simulink model "P1_DevDriv_z_krancowka_2015a"  (R2020b)
settings: Solver=ode5  StartTime=0.0  StopTime=999  FixedStep=0.01  RelTol=1e-3  AbsTol=1e-6
undefined symbols (not defined in the file): Cntrl, K_reg, RTDAC4PCIBaseAddress, x_konc
libraries: simulink x2
settings Model: SimulationMode=external  ExtModeTrigDuration=12000  ExtModeTrigDurationFloating=999000  ExtModeTrigLevel=0.400000  Creator=jims  LastModifiedBy=maelstro
settings SolverCC: AutoScaleAbsTol=off
settings DataIOCC: ExternalInput=[]  InitialState=[]  MaxDataPoints=5000  SaveFormat=Array  SignalLoggingSaveFormat=ModelDataLogs  SaveOutput=off  SaveTime=off  ReturnWorkspaceOutputs=off  SignalLoggingName=sigsOut
settings OptimizationCC: BooleanDataType=off  ExpressionDepthLimit=2147483647  LifeSpan=inf
settings DebuggingCC: SaveWithParameterizedLinksMsg=none  UnderspecifiedInitializationDetection=Classic  MergeDetectMultiDrivingBlocksExec=none  SignalResolutionControl=TryResolveAllWithWarning  MultiTaskDSMMsg=warning  MultiTaskCondExecSysMsg=none  IntegerOverflowMsg=none  FcnCallInpInsideContextMsg=warning  StateNameClashWarn=warning  SFUnexpectedBacktrackingDiag=warning  SFNoUnconditionalDefaultTransitionDiag=warning  SFExecutionAtInitializationDiag=none  IntegerSaturationMsg=none  ArithmeticOperatorsInVariantConditions=warning
settings HardwareCC: ProdBitPerLong=64  ProdLargestAtomicFloat=None  ProdHWDeviceType=Intel->x86-64  TargetBitPerLong=64  TargetBitPerPointer=64  TargetIntDivRoundTo=Zero  TargetEndianess=LittleEndian  TargetWordSize=64  TargetHWDeviceType=Intel->x86-64
settings ModelReferenceCC: PropagateSignalLabelsOutOfModel=off
settings SFSimCC: SimUseLocalCustomCode=off  CustomCodeUndefinedFunction=UseInterfaceOnly
settings RTWCC: Description=Real-Time Windows Target  SystemTargetFile=rtwin.tlc  TemplateMakefile=rtwin.tmf  RTWUseLocalCustomCode=off  RTWCompilerOptimization=on
settings CodeAppCC: MaxIdLength=95  StateflowObjectComments=on
settings TargetCC: TargetPreCompLibLocation=C:\Program Files\MATLAB\R2015aSP1\toolbox\sldrt\lib\win64
settings ConfigComp: CovMetricSettings=dw  CovSaveCumulativeToWorkspaceVar=on  CovSaveSingleToWorkspaceVar=on  CovExternalEMLEnable=off  CovSFcnEnable=off

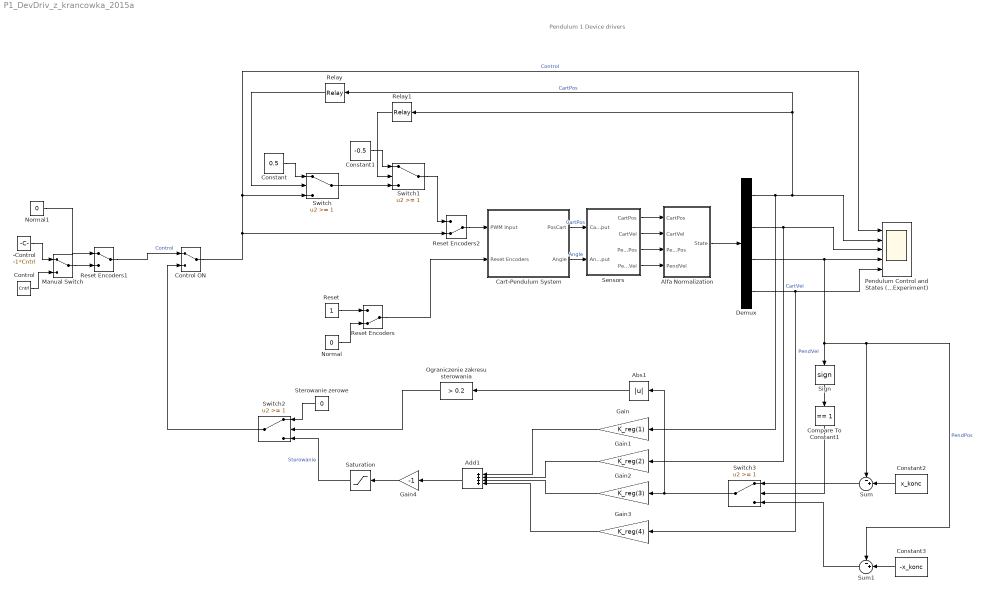
== system P1_DevDriv_z_krancowka_2015a ==
  note: Pendulum 1
      | Device drivers
  -Control : Constant  Value=-1*Cntrl
  Abs1 : Abs
  Add1 : Sum  Inputs=++++
  Alfa Normalization : Subsystem  mask(Choose mode:){pos=Crane Controller}
      mask prompts: pos "Choose mode:"
      mask TypeOptions pos: Inverted Pendulum | Crane Controller
  Cart-Pendulum System : Subsystem  mask{BaseAddress=RTDAC4PCIBaseAddress(-1,-1), T0=0.01}
      mask prompts: BaseAddress "Base Address:"; T0 "Sampling Period:"
      mask Display: plot( [0.725 0.725], [1.05 0.375], 0.725+0.05*sin([0:0.5:7]), 0.325+0.05*cos([0:0.5:7]), [-0.3 -0.3], [-0.3 -0.3], [1.8 1.8], [1.8 1.8], [0.1 1.4], [0.95 0.95], [0.1 1.4], [0.92 0.92], [0.65 0.8], [1 1], [0.65 0.8], [1.1 1.1], [0.65 0.65], [1.1 1], [0.8 0.8], [1 1.1] )
  Compare To Constant1 : simulink/Logic and Bit Operations/Compare To Constant  relop===  const=1  OutDataTypeStr=boolean
  Constant : Constant  Value=0.5
  Constant1 : Constant  Value=-0.5
  Constant2 : Constant  Value=x_konc
  Constant3 : Constant  Value=-x_konc
  Control : Constant  Value=Cntrl
  Control ON : ManualSwitch
  Demux : Demux
      settings: DisplayOption=none
  Gain : Gain  Gain=K_reg(1)
  Gain1 : Gain  Gain=K_reg(2)
  Gain2 : Gain  Gain=K_reg(3)
  Gain3 : Gain  Gain=K_reg(4)
  Gain4 : Gain  Gain=-1
  Manual Switch : ManualSwitch
  Normal : Constant  Value=0
  Normal1 : Constant  Value=0
  Ograniczenie zakresu sterowania : simulink/Logic and Bit Operations/Compare To Constant  relop=>  const=0.2  OutDataTypeStr=boolean
  Pendulum Control and States (Experiment) : Scope  NumInputPorts=5
  Relay : Relay  OnSwitchValue=0.7  OffSwitchValue=0.6
  Relay1 : Relay  OnSwitchValue=-0.6  OffSwitchValue=-0.7  OnOutputValue=0  OffOutputValue=1
  Reset : Constant
  Reset Encoders : ManualSwitch  CurrentSetting=0
  Reset Encoders1 : ManualSwitch
  Reset Encoders2 : ManualSwitch  CurrentSetting=0
  Saturation : Saturate  UpperLimit=1  LowerLimit=-1
  Sensors : Subsystem  mask(PENDULUM Output){T0=0.01}
      mask prompts: T0 "Sample Time"
      mask help: PCL-812 PG Device Driver
  Sign : Signum
  Sterowanie zerowe : Constant  Value=0
  Sum : Sum  Inputs=-+|
  Sum1 : Sum  Inputs=-+|
  Switch{,1..3} (4 alike) : Switch  Threshold=1
  wires:
  Reset Encoders/1 -> Cart-Pendulum System/2(Reset Encoders)
  Sensors/3(PendPos) -> Alfa Normalization/3(PendPos)
  Sensors/4(PendVel) -> Alfa Normalization/4(PendVel)
  Sensors/1(CartPos) -> Alfa Normalization/1(CartPos)
  Sensors/2(CartVel) -> Alfa Normalization/2(CartVel)
  Demux/1 -> Gain/1, Pendulum Control and States (Experiment)/2, Relay/1, Relay1/1  "CartPos"
  Demux/2 -> Gain1/1, Pendulum Control and States (Experiment)/3  "CartVel"
  Demux/3 -> Sum1/1, Sum/1, Sign/1, Pendulum Control and States (Experiment)/4  "PendPos"
  Demux/4 -> Gain3/1, Pendulum Control and States (Experiment)/5  "PendVel"
  Cart-Pendulum System/1(PosCart) -> Sensors/1(CartPosInput)  "CartPos"
  Cart-Pendulum System/2(Angle) -> Sensors/2(AngleInput)  "Angle"
  Normal/1 -> Reset Encoders/2
  Reset/1 -> Reset Encoders/1
  Normal1/1 -> Reset Encoders1/1
  Manual Switch/1 -> Reset Encoders1/2
  Control/1 -> Manual Switch/2
  -Control/1 -> Manual Switch/1
  Control ON/1 -> Reset Encoders2/2, Pendulum Control and States (Experiment)/1, Switch/3  "Control"
  Relay/1 -> Switch/2
  Constant/1 -> Switch/1
  Reset Encoders2/1 -> Cart-Pendulum System/1(PWM Input)
  Relay1/1 -> Switch1/2
  Constant1/1 -> Switch1/1
  Switch/1 -> Switch1/3
  Switch1/1 -> Reset Encoders2/1
  Gain/1 -> Add1/1
  Gain1/1 -> Add1/2
  Gain2/1 -> Add1/3
  Gain3/1 -> Add1/4
  Constant2/1 -> Sum/2
  Add1/1 -> Gain4/1
  Gain4/1 -> Saturation/1
  Reset Encoders1/1 -> Control ON/1  "Control"
  Abs1/1 -> Ograniczenie zakresu sterowania/1
  Ograniczenie zakresu sterowania/1 -> Switch2/2
  Sterowanie zerowe/1 -> Switch2/1
  Saturation/1 -> Switch2/3  "Sterowanie"
  Switch2/1 -> Control ON/2
  Constant3/1 -> Sum1/2
  Sign/1 -> Compare To Constant1/1
  Compare To Constant1/1 -> Switch3/2
  Sum/1 -> Switch3/1
  Sum1/1 -> Switch3/3
  Alfa Normalization/1(State) -> Demux/1
  Switch3/1 -> Gain2/1, Abs1/1

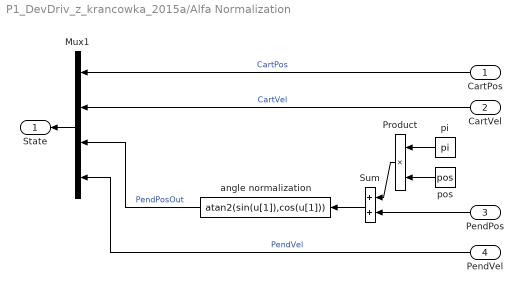
== system P1_DevDriv_z_krancowka_2015a/Alfa Normalization ==
  CartPos : Inport
  CartVel : Inport  Port=2
  PendPos : Inport  Port=3
  PendVel : Inport  Port=4
  Mux1 : Mux
  Product : Product  InputSameDT=on  SaturateOnIntegerOverflow=on  OutDataTypeStr=Inherit: Same as first input
  Sum : Sum  InputSameDT=on  SaturateOnIntegerOverflow=on  OutDataTypeStr=Inherit: Same as first input
  angle normalization : Fcn  Expr=atan2(sin(u[1]),cos(u[1]))
  pi : Constant  Value=pi
  pos : Constant  Value=pos
  State : Outport  InitialOutput=0
  wires:
  angle normalization/1 -> Mux1/3  "PendPosOut"
  PendVel/1 -> Mux1/4  "PendVel"
  CartVel/1 -> Mux1/2  "CartVel"
  CartPos/1 -> Mux1/1  "CartPos"
  Mux1/1 -> State/1
  Sum/1 -> angle normalization/1
  PendPos/1 -> Sum/2
  pi/1 -> Product/1
  pos/1 -> Product/2
  Product/1 -> Sum/1

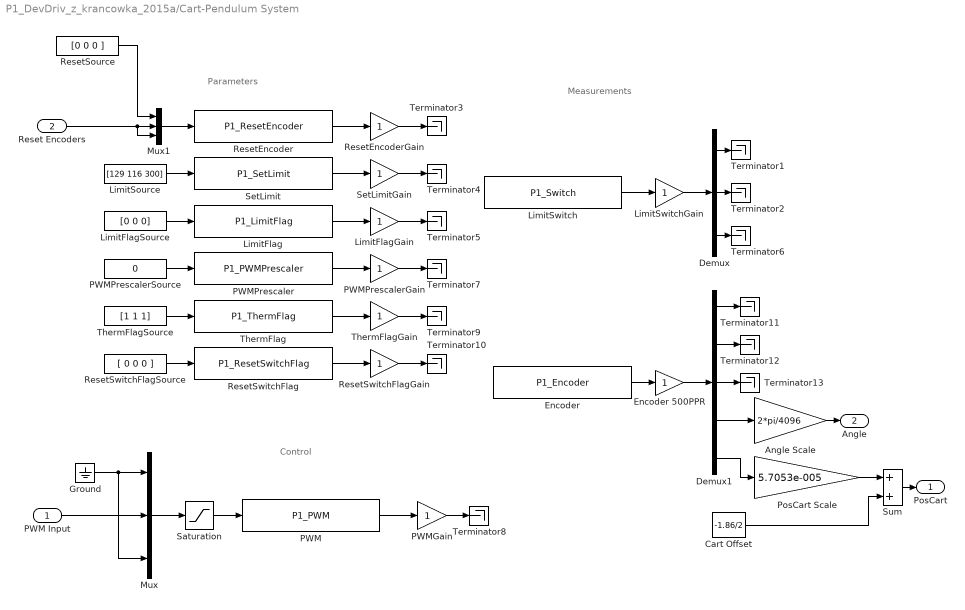
== system P1_DevDriv_z_krancowka_2015a/Cart-Pendulum System ==
  note: Measurements
  note: Control
  note: Parameters
  PWM Input : Inport
  Reset Encoders : Inport  Port=2
  Angle Scale : Gain  Gain=2*pi/4096  OutDataTypeStr=Inherit: Same as input  ParamDataTypeStr=Inherit: Same as input
  Cart Offset : Constant  Value=-1.86/2
  Demux : Demux  Outputs=3
      settings: DisplayOption=none
  Demux1 : Demux  Outputs=5
      settings: DisplayOption=none
  Encoder : S-Function  FunctionName=P1_Encoder  Parameters=BaseAddress, T0  SFunctionDeploymentMode=off  EnableBusSupport=off
  Encoder 500PPR : Gain  SaturateOnIntegerOverflow=on  OutDataTypeStr=Inherit: Same as input  ParamDataTypeStr=Inherit: Same as input
  Ground : Ground
  LimitFlag : S-Function  FunctionName=P1_LimitFlag  Parameters=BaseAddress, T0  SFunctionDeploymentMode=off  EnableBusSupport=off
  LimitFlagGain : Gain  SaturateOnIntegerOverflow=on  OutDataTypeStr=Inherit: Same as input  ParamDataTypeStr=Inherit: Same as input
  LimitFlagSource : Constant  Value=[0 0 0]
  LimitSource : Constant  Value=[129 116 300]
  LimitSwitch : S-Function  FunctionName=P1_Switch  Parameters=BaseAddress, T0  SFunctionDeploymentMode=off  EnableBusSupport=off
  LimitSwitchGain : Gain  SaturateOnIntegerOverflow=on  OutDataTypeStr=Inherit: Same as input  ParamDataTypeStr=Inherit: Same as input
  Mux : Mux  Inputs=3
  Mux1 : Mux  Inputs=[3 1 1]
  PWM : S-Function  FunctionName=P1_PWM  Parameters=BaseAddress, T0  SFunctionDeploymentMode=off  EnableBusSupport=off
  PWMGain : Gain  SaturateOnIntegerOverflow=on  OutDataTypeStr=Inherit: Same as input  ParamDataTypeStr=Inherit: Same as input
  PWMPrescaler : S-Function  FunctionName=P1_PWMPrescaler  Parameters=BaseAddress, T0  SFunctionDeploymentMode=off  EnableBusSupport=off
  PWMPrescalerGain : Gain  SaturateOnIntegerOverflow=on  OutDataTypeStr=Inherit: Same as input  ParamDataTypeStr=Inherit: Same as input
  PWMPrescalerSource : Constant  Value=0
  PosCart Scale : Gain  Gain=5.7053e-005  OutDataTypeStr=Inherit: Same as input  ParamDataTypeStr=Inherit: Same as input
  ResetEncoder : S-Function  FunctionName=P1_ResetEncoder  Parameters=BaseAddress, T0  SFunctionDeploymentMode=off  EnableBusSupport=off
  ResetEncoderGain : Gain  SaturateOnIntegerOverflow=on  OutDataTypeStr=Inherit: Same as input  ParamDataTypeStr=Inherit: Same as input
  ResetSource : Constant  Value=[0 0 0 ]
  "ResetSwitchFlag " : S-Function  FunctionName=P1_ResetSwitchFlag  Parameters=BaseAddress, T0  SFunctionDeploymentMode=off  EnableBusSupport=off
  ResetSwitchFlagGain : Gain  SaturateOnIntegerOverflow=on  OutDataTypeStr=Inherit: Same as input  ParamDataTypeStr=Inherit: Same as input
  ResetSwitchFlagSource : Constant  Value=[ 0 0 0 ]
  Saturation : Saturate
  SetLimit : S-Function  FunctionName=P1_SetLimit  Parameters=BaseAddress, T0  SFunctionDeploymentMode=off  EnableBusSupport=off
  SetLimitGain : Gain  SaturateOnIntegerOverflow=on  OutDataTypeStr=Inherit: Same as input  ParamDataTypeStr=Inherit: Same as input
  Sum : Sum  InputSameDT=on  SaturateOnIntegerOverflow=on  OutDataTypeStr=Inherit: Same as first input
  Terminator{1..13} (13 alike) : Terminator
  "ThermFlag " : S-Function  FunctionName=P1_ThermFlag  Parameters=BaseAddress, T0  SFunctionDeploymentMode=off  EnableBusSupport=off
  ThermFlagGain : Gain  SaturateOnIntegerOverflow=on  OutDataTypeStr=Inherit: Same as input  ParamDataTypeStr=Inherit: Same as input
  ThermFlagSource : Constant  Value=[1 1 1]
  PosCart : Outport  InitialOutput=0
  Angle : Outport  Port=2  InitialOutput=0
  wires:
  Demux1/1 -> Terminator11/1
  Demux1/2 -> Terminator12/1
  Demux1/3 -> Terminator13/1
  Demux1/4 -> Angle Scale/1
  Demux1/5 -> PosCart Scale/1
  Angle Scale/1 -> Angle/1
  Demux/3 -> Terminator6/1
  Demux/2 -> Terminator2/1
  Demux/1 -> Terminator1/1
  LimitSwitchGain/1 -> Demux/1
  LimitSwitch/1 -> LimitSwitchGain/1
  Ground/1 -> Mux/1, Mux/3
  PWM Input/1 -> Mux/2
  ResetSwitchFlagGain/1 -> Terminator10/1
  ThermFlagGain/1 -> Terminator9/1
  PWMPrescalerGain/1 -> Terminator7/1
  LimitFlagGain/1 -> Terminator5/1
  SetLimitGain/1 -> Terminator4/1
  ResetEncoderGain/1 -> Terminator3/1
  ResetSwitchFlagSource/1 -> "ResetSwitchFlag "/1
  ThermFlagSource/1 -> "ThermFlag "/1
  PWMPrescalerSource/1 -> PWMPrescaler/1
  LimitFlagSource/1 -> LimitFlag/1
  LimitSource/1 -> SetLimit/1
  "ResetSwitchFlag "/1 -> ResetSwitchFlagGain/1
  "ThermFlag "/1 -> ThermFlagGain/1
  PWMPrescaler/1 -> PWMPrescalerGain/1
  LimitFlag/1 -> LimitFlagGain/1
  SetLimit/1 -> SetLimitGain/1
  ResetEncoder/1 -> ResetEncoderGain/1
  PWMGain/1 -> Terminator8/1
  PWM/1 -> PWMGain/1
  Mux/1 -> Saturation/1
  Saturation/1 -> PWM/1
  Encoder/1 -> Encoder 500PPR/1
  Encoder 500PPR/1 -> Demux1/1
  Mux1/1 -> ResetEncoder/1
  ResetSource/1 -> Mux1/1
  Reset Encoders/1 -> Mux1/2, Mux1/3
  PosCart Scale/1 -> Sum/1
  Sum/1 -> PosCart/1
  Cart Offset/1 -> Sum/2

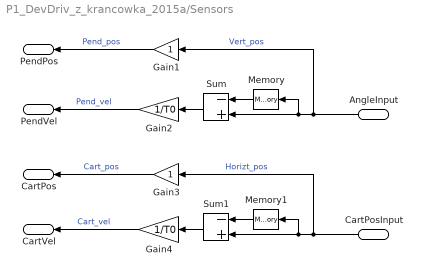
== system P1_DevDriv_z_krancowka_2015a/Sensors ==
  CartPosInput : Inport
  AngleInput : Inport  Port=2
  Gain1 : Gain  SaturateOnIntegerOverflow=on  OutDataTypeStr=Inherit: Same as input  ParamDataTypeStr=Inherit: Same as input
  Gain2 : Gain  Gain=1/T0  SaturateOnIntegerOverflow=on  OutDataTypeStr=Inherit: Same as input  ParamDataTypeStr=Inherit: Same as input
  Gain3 : Gain  SaturateOnIntegerOverflow=on  OutDataTypeStr=Inherit: Same as input  ParamDataTypeStr=Inherit: Same as input
  Gain4 : Gain  Gain=1/T0  SaturateOnIntegerOverflow=on  OutDataTypeStr=Inherit: Same as input  ParamDataTypeStr=Inherit: Same as input
  Memory : Memory
  Memory1 : Memory
  Sum : Sum  Inputs=-+  InputSameDT=on  SaturateOnIntegerOverflow=on  OutDataTypeStr=Inherit: Same as first input
  Sum1 : Sum  Inputs=-+  InputSameDT=on  SaturateOnIntegerOverflow=on  OutDataTypeStr=Inherit: Same as first input
  CartPos : Outport  InitialOutput=0
  CartVel : Outport  Port=2  InitialOutput=0
  PendPos : Outport  Port=3  InitialOutput=0
  PendVel : Outport  Port=4  InitialOutput=0
  wires:
  Gain4/1 -> CartVel/1  "Cart_vel"
  Sum1/1 -> Gain4/1
  Memory1/1 -> Sum1/1
  Sum/1 -> Gain2/1
  Memory/1 -> Sum/1
  CartPosInput/1 -> Memory1/1, Sum1/2, Gain3/1  "Horizt_pos"
  AngleInput/1 -> Memory/1, Sum/2, Gain1/1  "Vert_pos"
  Gain2/1 -> PendVel/1  "Pend_vel"
  Gain1/1 -> PendPos/1  "Pend_pos"
  Gain3/1 -> CartPos/1  "Cart_pos"
